simulink model "Sim_Multi"  (R2019b)
settings: Solver=VariableStepAuto  StartTime=0.0  StopTime=sim_time  FixedStep=t_sim  MaxStep=t_control  RelTol=1e-5  EnableMultiTasking=on
model workspace (MAT data in the model file):
  start_time = 1
values from neighbouring files (symbols this model uses):
  Att_init = [0;0;0] * d2r    [Init_Multi.m]
  Blade_flapping = 0    [Init_Multi.m]
  C_D = 0.40    (= 0.4)    [Init_Multi.m]
  CoG_nominal = [0;0;0.001]    [Init_Multi.m]
  CoG_real = [0;0;0.001]    [Init_Multi.m]
  Coriolis_correction = 0    [Init_Multi.m]
  d2r = pi/180    (= 0.0174532925199)    [Init_Multi.m]
  Dyn_thrust = 0    [Init_Multi.m]
  g = 9.80665    [Init_Multi.m]
  J_nominal = [Jxx Jxy Jxz;Jyx Jyy Jyz;Jzx Jzy Jzz]    [Init_Multi.m]
  J_real = [Jxx Jxy Jxz;Jyx Jyy Jyz;Jzx Jzy Jzz]    [Init_Multi.m]
  k1 = -1.125    [Init_Multi.m]
  k2 = -1.372    [Init_Multi.m]
  k3 = -1.718    [Init_Multi.m]
  k4 = -0.655    [Init_Multi.m]
  k_a1s = 1.5 / 4.0    (= 0.375)    [Init_Multi.m]
  k_beta = 0.23    [Init_Multi.m]
  kappa = 1.00    (= 1)    [Init_Multi.m]
  mass_nominal = 0.550    (= 0.55)    [Init_Multi.m]
  mass_real = 0.550    (= 0.55)    [Init_Multi.m]
  max_thrust = max_thrust + (MotorMatrix_nominal(i,7)*MotorMatrix_nominal(i,12)+MotorMatrix_nominal(i,8)*MotorMatrix_nominal(i,12)^2)    [Init_Multi.m]
  MaxRate_cmd = [360;360;120] * d2r    [Init_Multi.m]
  min_thrust = min_thrust + (MotorMatrix_nominal(i,7)*MotorMatrix_nominal(i,11)+MotorMatrix_nominal(i,8)*MotorMatrix_nominal(i,11)^2)    [Init_Multi.m]
  MotorMap = B' * inv(B * B')    [Init_Multi.m]
  MotorMatrix_nominal = [045 , 0.170 , -0.028 , -1 , 1.0 , 0.010 , [9.6820 , 0.010872]*1e-5 , [1.4504 , 0.0016312]*1e-6 , 0000 , 6000 , [0.0 , 0.0 , 0.0] , 8*2.54/100 , 11/1000;                         135 , 0.170 , -0.028 , +1 , 1.0 , 0.010 , [9.6820 , 0.010872]*1e-5 , [1.4504 , 0.0016312]*1e-6 , 0000 , 6000 , [0.0 , 0.0 , 0.0] , 8*2.54/100 , 11/1000;                         225 , 0.170 , -0.028 , -1 , 1.0 , 0.010 , [9. ...(+284 chars)    [Init_Multi.m]
  MotorMatrix_real = [045 , 0.170 , -0.028 , -1 , 1.0 , 0.010 , [9.6820 , 0.010872]*1e-5 , [1.4504 , 0.0016312]*1e-6 , 0000 , 6000 , [0.0 , 0.0 , 0.0] , 8*2.54/100 , 11/1000;                      135 , 0.170 , -0.028 , +1 , 1.0 , 0.010 , [9.6820 , 0.010872]*1e-5 , [1.4504 , 0.0016312]*1e-6 , 0000 , 6000 , [0.0 , 0.0 , 0.0] , 8*2.54/100 , 11/1000;                      225 , 0.170 , -0.028 , -1 , 1.0 , 0.010 , [9.6820 , ...(+275 chars)    [Init_Multi.m]
  Noise_flag = 1    [Init_Multi.m]
  omega_init = [0;0;0]    [Init_Multi.m]
  q_init = rpy2quat(Att_init)    [Init_Multi.m]
  r2d = 180/pi    (= 57.2957795131)    [Init_Multi.m]
  rho = 1.225    [Init_Multi.m]
  rpm2radpersec = 2*pi/60    (= 0.10471975512)    [Init_Multi.m]
  rpm_init = 3104.5025852    [Init_Multi.m]
  Surface_params = [a;b;c]    [Init_Multi.m]
  t_control = t_control_2*4    (= 0.02)    [Init_Multi.m]
  t_sim = 1/1000    (= 0.001)    [Init_Multi.m]
  thrust_reserve = 0.10    (= 0.1)    [Init_Multi.m]
  v_h = 4.0    (= 4)    [Init_Multi.m]
  Vb_init = [0;0;0]    [Init_Multi.m]
  Vi_init = R_IB_init' * Vb_init    [Init_Multi.m]
  Xi_init = [0;0;-1]    [Init_Multi.m]
undefined symbols (not defined in the file or in its folder): anti_windup_1, anti_windup_2, DiscIntNeverNeededParam, Kd_1, Kd_2, Kff_1, Kff_2, Ki_1, Ki_2, Kp_1, Kp_2, Kpass_1, magnitude, rpy2quat, thrust2rpm
libraries: simulink x35, dspsigops x3, sharedtransform x2, dspmtrx3 x1, robotuavlib x1, vrlib x1
(part 3 of 4)

== system Sim_Multi/Controller/Controller Structure/Pos//Vel Control/PI Rate controller1/Gain Kff ==
  Rate_cmd : Inport
  Constant1 : Constant  Value=Kff_1
  Create diagonal 3x3 matrix : Subsystem
  Product : Product  Multiplication=Matrix(*)  SampleTime=t_control  RndMeth=Zero
  Product1 : Product  Multiplication=Matrix(*)  RndMeth=Zero
  Out1 : Outport
  wires:
  [J_control] -> Product1/1
  Product1/1 -> Product/1
  Rate_cmd/1 -> Product/2
  Constant1/1 -> Create diagonal 3x3 matrix/1(Vector)
  Create diagonal 3x3 matrix/1(Matrix) -> Product1/2
  Product/1 -> Out1/1

== system Sim_Multi/Controller/Controller Structure/Pos//Vel Control/PI Rate controller1/Gain Ki ==
  Rate_error : Inport
  Constant1 : Constant  Value=Ki_1
  Create diagonal 3x3 matrix : Subsystem
  Product : Product  Multiplication=Matrix(*)  SampleTime=t_control  RndMeth=Zero
  Product1 : Product  Multiplication=Matrix(*)  RndMeth=Zero
  Out1 : Outport
  wires:
  [J_control] -> Product1/1
  Product1/1 -> Product/1
  Rate_error/1 -> Product/2
  Constant1/1 -> Create diagonal 3x3 matrix/1(Vector)
  Create diagonal 3x3 matrix/1(Matrix) -> Product1/2
  Product/1 -> Out1/1

== system Sim_Multi/Controller/Controller Structure/Pos//Vel Control/PI Rate controller1/Gain Kp ==
  Rate_error : Inport
  Constant1 : Constant  Value=Kp_1
  Create diagonal 3x3 matrix : Subsystem
  Product : Product  Multiplication=Matrix(*)  SampleTime=t_control  RndMeth=Zero
  Product1 : Product  Multiplication=Matrix(*)  RndMeth=Zero
  Out1 : Outport
  wires:
  [J_control] -> Product1/1
  Product1/1 -> Product/1
  Rate_error/1 -> Product/2
  Constant1/1 -> Create diagonal 3x3 matrix/1(Vector)
  Create diagonal 3x3 matrix/1(Matrix) -> Product1/2
  Product/1 -> Out1/1

== system Sim_Multi/Controller/Controller Structure/Pos//Vel Control/PID Attitude Controller (additionally controls altitude and yaw to take advantage of faster sampling rate)1/Gain Kd ==
  Rate_error : Inport
  Constant1 : Constant  Value=Kd_2
  Product : Product  RndMeth=Zero
  Out1 : Outport
  wires:
  Rate_error/1 -> Product/2
  Product/1 -> Out1/1
  Constant1/1 -> Product/1

== system Sim_Multi/Controller/Controller Structure/Pos//Vel Control/PID Attitude Controller (additionally controls altitude and yaw to take advantage of faster sampling rate)1/Gain Ki ==
  Rate_error : Inport
  Constant1 : Constant  Value=Ki_2
  Product : Product  RndMeth=Zero
  Out1 : Outport
  wires:
  Rate_error/1 -> Product/2
  Product/1 -> Out1/1
  Constant1/1 -> Product/1

== system Sim_Multi/Controller/Controller Structure/Pos//Vel Control/PID Attitude Controller (additionally controls altitude and yaw to take advantage of faster sampling rate)1/Gain Kp ==
  Rate_error : Inport
  Constant1 : Constant  Value=Kp_2
  Product : Product  RndMeth=Zero
  Out1 : Outport
  wires:
  Rate_error/1 -> Product/2
  Product/1 -> Out1/1
  Constant1/1 -> Product/1

== system Sim_Multi/Controller/Controller Structure/Pos//Vel Control/PID Position Controller (yaw and Z are passed though)1/Gain Kd ==
  Rate_error : Inport
  Constant1 : Constant  Value=Kd_1
  Product : Product  SampleTime=t_control  RndMeth=Zero
  Out1 : Outport
  wires:
  Rate_error/1 -> Product/2
  Product/1 -> Out1/1
  Constant1/1 -> Product/1

== system Sim_Multi/Controller/Controller Structure/Pos//Vel Control/PID Position Controller (yaw and Z are passed though)1/Gain Ki ==
  Rate_error : Inport
  Constant1 : Constant  Value=Ki_1
  Product : Product  SampleTime=t_control  RndMeth=Zero
  Out1 : Outport
  wires:
  Rate_error/1 -> Product/2
  Product/1 -> Out1/1
  Constant1/1 -> Product/1

== system Sim_Multi/Controller/Controller Structure/Pos//Vel Control/PID Position Controller (yaw and Z are passed though)1/Gain Kp ==
  Rate_error : Inport
  Constant1 : Constant  Value=Kp_1
  Product : Product  SampleTime=t_control  RndMeth=Zero
  Out1 : Outport
  wires:
  Rate_error/1 -> Product/2
  Product/1 -> Out1/1
  Constant1/1 -> Product/1

== system Sim_Multi/Plant/6DOF model/Calculate omega_dot/Cross Product omega x (J * omega)/Subsystem ==
  u : Inport
  v : Inport  Port=2
  Demux : Demux  Outputs=3
  Demux1 : Demux  Outputs=3
  Mux : Mux  Inputs=3
  Product : Product
  Product1 : Product
  Product2 : Product
  Positive elements : Outport
  wires:
  Mux/1 -> Positive elements/1
  v/1 -> Demux1/1
  u/1 -> Demux/1
  Demux/2 -> Product/1
  Demux1/3 -> Product/2
  Demux/3 -> Product1/1
  Demux1/1 -> Product1/2
  Demux/1 -> Product2/1
  Demux1/2 -> Product2/2
  Product/1 -> Mux/1  "u2*v3"
  Product1/1 -> Mux/2  "u3*v1"
  Product2/1 -> Mux/3  "u1*v2"

== system Sim_Multi/Plant/6DOF model/Calculate omega_dot/Cross Product omega x (J * omega)/Subsystem1 ==
  u : Inport
  v : Inport  Port=2
  Demux : Demux  Outputs=3
  Demux1 : Demux  Outputs=3
  Mux : Mux  Inputs=3
  Product : Product
  Product1 : Product
  Product2 : Product
  Negative elements : Outport
  wires:
  Mux/1 -> Negative elements/1
  v/1 -> Demux1/1
  u/1 -> Demux/1
  Product/1 -> Mux/1  "u3*v2"
  Product1/1 -> Mux/2  "u1*v3"
  Product2/1 -> Mux/3  "u2*v1"
  Demux/3 -> Product/1
  Demux1/2 -> Product/2
  Demux/1 -> Product1/1
  Demux1/3 -> Product1/2
  Demux/2 -> Product2/1
  Demux1/1 -> Product2/2

== system Sim_Multi/Plant/6DOF model/Quat Strapdown Eq./Cross Product/Subsystem ==
  u : Inport
  v : Inport  Port=2
  Demux : Demux  Outputs=3
  Demux1 : Demux  Outputs=3
  Mux : Mux  Inputs=3
  Product : Product
  Product1 : Product
  Product2 : Product
  Positive elements : Outport
  wires:
  Mux/1 -> Positive elements/1
  v/1 -> Demux1/1
  u/1 -> Demux/1
  Demux/2 -> Product/1
  Demux1/3 -> Product/2
  Demux/3 -> Product1/1
  Demux1/1 -> Product1/2
  Demux/1 -> Product2/1
  Demux1/2 -> Product2/2
  Product/1 -> Mux/1  "u2*v3"
  Product1/1 -> Mux/2  "u3*v1"
  Product2/1 -> Mux/3  "u1*v2"

== system Sim_Multi/Plant/6DOF model/Quat Strapdown Eq./Cross Product/Subsystem1 ==
  u : Inport
  v : Inport  Port=2
  Demux : Demux  Outputs=3
  Demux1 : Demux  Outputs=3
  Mux : Mux  Inputs=3
  Product : Product
  Product1 : Product
  Product2 : Product
  Negative elements : Outport
  wires:
  Mux/1 -> Negative elements/1
  v/1 -> Demux1/1
  u/1 -> Demux/1
  Product/1 -> Mux/1  "u3*v2"
  Product1/1 -> Mux/2  "u1*v3"
  Product2/1 -> Mux/3  "u2*v1"
  Demux/3 -> Product/1
  Demux1/2 -> Product/2
  Demux/1 -> Product1/1
  Demux1/3 -> Product1/2
  Demux/2 -> Product2/1
  Demux1/1 -> Product2/2

== system Sim_Multi/Plant/6DOF model/Quat Strapdown Eq./Normalize/norm ==
  u : Inport
  Complex to Real-Imag : ComplexToRealImag  Output=Real
  Sqrt : Sqrt  SaturateOnIntegerOverflow=on
  dot_product : Subsystem
  ||u|| : Outport
  wires:
  u/1 -> dot_product/1(u), dot_product/2(v)
  dot_product/1(u.v) -> Sqrt/1
  Sqrt/1 -> Complex to Real-Imag/1
  Complex to Real-Imag/1 -> ||u||/1

== system Sim_Multi/Plant/Force//Moment computation/Compute aerodynamic drag of the airframe in Body axes/Aerodynamic drag force/Nonzero airspeed ==
  Airspeed (Body) : Inport
  Surface_params : Inport  Port=2
  Action Port : ActionPort  ActionPortLabel=else
  Abs : Abs
  Constant : Constant  Value=1/2
  Constant1 : Constant  Value=rho
  Constant2 : Constant  Value=C_D
  Drag force opposes direction of airspeed : Gain  Gain=-1
  Normalize : Subsystem
  Product : Product  Inputs=5
  Product1 : Product
  Surface area computation : Subsystem
  u^2 : Subsystem
  Drag force : Outport
  wires:
  Airspeed (Body)/1 -> Surface area computation/1(Airspeed (Body)), Normalize/1(Input), u^2/1(u)
  Surface_params/1 -> Surface area computation/2(Surface_params)
  Constant/1 -> Product/1
  Constant1/1 -> Product/2
  u^2/1(u^2) -> Product/3
  Constant2/1 -> Product/4
  Surface area computation/1(Area) -> Product/5
  Normalize/1(Output) -> Product1/1  "Normalized airspeed vector (Body axes)"
  Product1/1 -> Drag force opposes direction of airspeed/1
  Drag force opposes direction of airspeed/1 -> Drag force/1
  Product/1 -> Abs/1
  Abs/1 -> Product1/2  "Magnitude of drag force"

== system Sim_Multi/Plant/Force//Moment computation/Compute aerodynamic drag of the airframe in Body axes/Aerodynamic drag force/Zero airspeed ==
  Airspeed : Inport
  Surface_params : Inport  Port=2
  Action Port : ActionPort  ActionPortLabel=if(u1 == 0)
  Constant : Constant  Value=[0;0;0]
  Terminator : Terminator
  Terminator1 : Terminator
  Drag force : Outport  InitialOutput=[0;0;-1]
  wires:
  Airspeed/1 -> Terminator/1  "Airspeed components in (unbent) rotor plane"
  Constant/1 -> Drag force/1
  Surface_params/1 -> Terminator1/1

== system Sim_Multi/Plant/Force//Moment computation/Compute aerodynamic drag of the airframe in Body axes/Aerodynamic drag force/norm ==
  u : Inport
  Complex to Real-Imag : ComplexToRealImag  Output=Real
  Sqrt : Sqrt  SaturateOnIntegerOverflow=on
  dot_product : Subsystem
  ||u|| : Outport
  wires:
  u/1 -> dot_product/1(u), dot_product/2(v)
  dot_product/1(u.v) -> Sqrt/1
  Sqrt/1 -> Complex to Real-Imag/1
  Complex to Real-Imag/1 -> ||u||/1

== system Sim_Multi/Plant/Force//Moment computation/Compute aerodynamic drag of the airframe in Body axes/Total airspeed (Body axes)/Inertial to Body ==
  DCM_ib : Inport
  Wind_i : Inport  Port=2
  Product : Product  Multiplication=Matrix(*)
  Reshape : Reshape  OutputDimensionality=Column vector (2-D)
  Reshape1 : Reshape  OutputDimensionality=Column vector (2-D)
  Wind_b : Outport
  wires:
  Reshape/1 -> Product/2
  Product/1 -> Reshape1/1
  Reshape1/1 -> Wind_b/1
  Wind_i/1 -> Reshape/1
  DCM_ib/1 -> Product/1  "DCM_ib"

== system Sim_Multi/Plant/Force//Moment computation/Forces and moments generated by spinning propellers/For Each Subsystem/Actuator dynamics ==
  note: This block diagram expresses the actuator dynamics of a specific motor/propeller combination
      | as a first order transfer function. The time constant and gain of this first order transfer function
      | for each motor is listed in the motor matrix.
      | In addition, upper and lower limits of the motor RPM can be set so that the motor output
      | never exceeds those values.
  MotorMatrix_real : Inport
  RPM_command : Inport  Port=2
  Continuous Integrator with dynamic upper/lower limits : Subsystem
  Divide : Product  Inputs=*/
  Product : Product  SampleTime=t_sim  RndMeth=Zero
  Rate Transition : RateTransition  OutPortSampleTime=t_sim
  Selector : Selector  InputPortWidth=17  IndexOptions=Index vector (dialog)  Indices=[5]  OutputSizes=1
  Selector1 : Selector  InputPortWidth=17  IndexOptions=Index vector (dialog)  Indices=[6]  OutputSizes=1
  Selector2 : Selector  InputPortWidth=17  IndexOptions=Index vector (dialog)  Indices=[11]  OutputSizes=1
  Selector3 : Selector  InputPortWidth=17  IndexOptions=Index vector (dialog)  Indices=[12]  OutputSizes=1
  Sum1 : Sum  Inputs=-+|
  RPM_motor : Outport
  wires:
  Sum1/1 -> Divide/1
  Selector1/1 -> Divide/2  "TF time constant"
  Product/1 -> Sum1/2
  Selector/1 -> Product/2  "TF gain"
  RPM_command/1 -> Product/1
  MotorMatrix_real/1 -> Selector3/1, Selector2/1, Selector1/1, Selector/1
  Divide/1 -> Continuous Integrator with dynamic upper/lower limits/1(Integrator input)
  Continuous Integrator with dynamic upper/lower limits/1(Output) -> Rate Transition/1, Sum1/1
  Selector2/1 -> Continuous Integrator with dynamic upper/lower limits/2(Lower limit)  "RPM min value"
  Selector3/1 -> Continuous Integrator with dynamic upper/lower limits/3(Upper limit)  "RPM max value"
  Rate Transition/1 -> RPM_motor/1

== system Sim_Multi/Plant/Force//Moment computation/Forces and moments generated by spinning propellers/For Each Subsystem/Cross Product ==
  r : Inport
  omega : Inport  Port=2
  Reshape : Reshape  OutputDimensionality=Column vector (2-D)
  Subsystem : Subsystem
  Subsystem1 : Subsystem
  Sum : Sum  Inputs=+|-
  omega x r : Outport
  wires:
  Sum/1 -> Reshape/1
  omega/1 -> Subsystem1/1(omega), Subsystem/1(omega)
  r/1 -> Subsystem1/2(r), Subsystem/2(r)
  Subsystem/1(Positive elements) -> Sum/1
  Subsystem1/1(Negative elements) -> Sum/2
  Reshape/1 -> omega x r/1

== system Sim_Multi/Plant/Force//Moment computation/Forces and moments generated by spinning propellers/For Each Subsystem/Leverarm vector from real CoG to each propeller (Body axes) ==
  note: This subsystem computes the leverarm vector from the real center of gravity
      | of the airframe to each propeller.
      | This vector is necessary to compute the moment contributions of each propeller.
  MotorMatrix_real : Inport
  CoG_real : Inport  Port=2
  Abs : Abs
  Conversion deg to rad : Gain  Gain=d2r
  Mux : Mux  Inputs=2
  Mux2 : Mux  Inputs=2
  Product4 : Product
  Reshape : Reshape  OutputDimensionality=Column vector (2-D)
  Reshape1 : Reshape  OutputDimensionality=Column vector (2-D)
  Selector3 : Selector  InputPortWidth=17  IndexOptions=Index vector (dialog)  Indices=[1]  OutputSizes=1
  Selector4 : Selector  InputPortWidth=17  IndexOptions=Index vector (dialog)  Indices=[2]  OutputSizes=1
  Selector5 : Selector  InputPortWidth=17  IndexOptions=Index vector (dialog)  Indices=[3]  OutputSizes=1
  Subtract : Sum  Inputs=+-
  Trigonometric Function : Trigonometry
  Trigonometric Function1 : Trigonometry  Operator=cos
  Prop_vector : Outport
  wires:
  Selector3/1 -> Conversion deg to rad/1  "Motor arm angle"
  Selector4/1 -> Abs/1  "Motor arm length"
  Selector5/1 -> Mux2/2  "Propeller Z offset"
  Conversion deg to rad/1 -> Trigonometric Function/1, Trigonometric Function1/1
  Trigonometric Function1/1 -> Mux/1  "Motor arm x component"
  Trigonometric Function/1 -> Mux/2  "Motor arm y component"
  Mux/1 -> Product4/1
  Abs/1 -> Product4/2
  Product4/1 -> Mux2/1  "Motor location x/y vector"
  Mux2/1 -> Reshape/1
  CoG_real/1 -> Reshape1/1  "Location of real CoG w.r.t. geometric center (Body axes)"
  Reshape/1 -> Subtract/1  "Vector from geometric center to propeller (Body axes)"
  Reshape1/1 -> Subtract/2
  Subtract/1 -> Prop_vector/1  "Vector from real CoG to propeller (Body axes)"
  MotorMatrix_real/1 -> Selector5/1, Selector4/1, Selector3/1

== system Sim_Multi/Plant/Force//Moment computation/Forces and moments generated by spinning propellers/For Each Subsystem/Thrust//moment vector for each propeller (Body axes) ==
  Prop_vector : Inport
  True airspeed : Inport  Port=2
  Body_rates : Inport  Port=3
  MotorMatrix_real : Inport  Port=4
  RPM_motor : Inport  Port=5
  6 DOF : Inport  Port=6
  Add : Sum  Inputs=++++
  Compute dynamic motor thrust and moments : Subsystem
  Coordinate transformation Body to Motor axes : Subsystem
  Cross Product : Subsystem
  Reshape : Reshape  OutputDimensionality=Column vector (2-D)
  Thrust_vector (Body axes) : Outport
  Motor_moments (Body axes) : Outport  Port=2
  wires:
  MotorMatrix_real/1 -> Coordinate transformation Body to Motor axes/1(MotorMatrix_real), Compute dynamic motor thrust and moments/2(MotorMatrix_real)
  True airspeed/1 -> Coordinate transformation Body to Motor axes/2(Airspeed (Body axes))
  Coordinate transformation Body to Motor axes/2(Airspeed (Motor axes)) -> Compute dynamic motor thrust and moments/4(Airspeed (Motor axes))
  RPM_motor/1 -> Compute dynamic motor thrust and moments/1(RPM_motor)
  Body_rates/1 -> Compute dynamic motor thrust and moments/5(Body_rates)
  Compute dynamic motor thrust and moments/3(Gyro moment (Body axes)) -> Add/3  "Gyroscopic moments per motor (Body axes)"
  Compute dynamic motor thrust and moments/1(Induced motor moment (Body axes)) -> Add/1  "Induced motor moment at dynamic conditions (Body axes)"
  Add/1 -> Motor_moments (Body axes)/1
  Coordinate transformation Body to Motor axes/1(R_mb) -> Compute dynamic motor thrust and moments/3(R_mb)
  Compute dynamic motor thrust and moments/4(Thrust_vector (Body axes)) -> Thrust_vector (Body axes)/1, Cross Product/2(v)
  Compute dynamic motor thrust and moments/2(Motor hub moment (Body axes)) -> Add/2  "Moment induced in motor hub due to blade flapping (Body axes)"
  Cross Product/1(u x v) -> Reshape/1
  Prop_vector/1 -> Cross Product/1(u)
  Reshape/1 -> Add/4
  6 DOF/1 -> Compute dynamic motor thrust and moments/6(6 DOF)

== system Sim_Multi/Plant/Force//Moment computation/Forces and moments generated by spinning propellers/Total airspeed (Body axes)/Inertial to Body ==
  DCM_ib : Inport
  Wind_i : Inport  Port=2
  Product : Product  Multiplication=Matrix(*)
  Reshape : Reshape  OutputDimensionality=Column vector (2-D)
  Reshape1 : Reshape  OutputDimensionality=Column vector (2-D)
  Wind_b : Outport
  wires:
  Reshape/1 -> Product/2
  Product/1 -> Reshape1/1
  Reshape1/1 -> Wind_b/1
  Wind_i/1 -> Reshape/1
  DCM_ib/1 -> Product/1  "DCM_ib"

== system Sim_Multi/State Estimation, Sensors, Noise/State estimation/Normalize/norm/dot_product ==
  u : Inport
  v : Inport  Port=2
  Product : Product  Multiplication=Matrix(*)  RndMeth=Zero
  Reshape : Reshape  OutputDimensionality=Column vector (2-D)
  Reshape1 : Reshape  OutputDimensionality=Column vector (2-D)
  transpose : Math  Operator=transpose  SaturateOnIntegerOverflow=on
  u.v : Outport
  wires:
  v/1 -> Reshape1/1
  u/1 -> Reshape/1
  Reshape/1 -> transpose/1
  transpose/1 -> Product/1
  Reshape1/1 -> Product/2
  Product/1 -> u.v/1

== system Sim_Multi/State Estimation, Sensors, Noise/State estimation/Normalize1/norm/dot_product ==
  u : Inport
  v : Inport  Port=2
  Product : Product  Multiplication=Matrix(*)  RndMeth=Zero
  Reshape : Reshape  OutputDimensionality=Column vector (2-D)
  Reshape1 : Reshape  OutputDimensionality=Column vector (2-D)
  transpose : Math  Operator=transpose  SaturateOnIntegerOverflow=on
  u.v : Outport
  wires:
  v/1 -> Reshape1/1
  u/1 -> Reshape/1
  Reshape/1 -> transpose/1
  transpose/1 -> Product/1
  Reshape1/1 -> Product/2
  Product/1 -> u.v/1

== system Sim_Multi/Controller/Controller Structure/Pos//Vel Control/PI Rate controller1/Cross Product/Subsystem ==
  u : Inport
  v : Inport  Port=2
  Demux : Demux  Outputs=3
  Demux1 : Demux  Outputs=3
  Mux : Mux  Inputs=3
  Product : Product
  Product1 : Product
  Product2 : Product
  Positive elements : Outport
  wires:
  Mux/1 -> Positive elements/1
  v/1 -> Demux1/1
  u/1 -> Demux/1
  Demux/2 -> Product/1
  Demux1/3 -> Product/2
  Demux/3 -> Product1/1
  Demux1/1 -> Product1/2
  Demux/1 -> Product2/1
  Demux1/2 -> Product2/2
  Product/1 -> Mux/1
  Product1/1 -> Mux/2
  Product2/1 -> Mux/3

== system Sim_Multi/Controller/Controller Structure/Pos//Vel Control/PI Rate controller1/Cross Product/Subsystem1 ==
  u : Inport
  v : Inport  Port=2
  Demux : Demux  Outputs=3
  Demux1 : Demux  Outputs=3
  Mux : Mux  Inputs=3
  Product : Product
  Product1 : Product
  Product2 : Product
  Negative elements : Outport
  wires:
  Mux/1 -> Negative elements/1
  v/1 -> Demux1/1
  u/1 -> Demux/1
  Product/1 -> Mux/1
  Product1/1 -> Mux/2
  Product2/1 -> Mux/3
  Demux/3 -> Product/1
  Demux1/2 -> Product/2
  Demux/1 -> Product1/1
  Demux1/3 -> Product1/2
  Demux/2 -> Product2/1
  Demux1/1 -> Product2/2

== system Sim_Multi/Controller/Controller Structure/Pos//Vel Control/PI Rate controller1/Gain Kff/Create diagonal 3x3 matrix ==
  Vector : Inport
  Constant2 : Constant  Value=0
  Demux : Demux  Outputs=3
  Subsystem9 : Subsystem
  Matrix : Outport
  wires:
  Demux/1 -> Subsystem9/1(C_11)
  Demux/2 -> Subsystem9/5(C_22)
  Vector/1 -> Demux/1
  Constant2/1 -> Subsystem9/8(C_32), Subsystem9/7(C_31), Subsystem9/6(C_23), Subsystem9/4(C_21), Subsystem9/3(C_13), Subsystem9/2(C_12)
  Subsystem9/1(Diag) -> Matrix/1
  Demux/3 -> Subsystem9/9(C_33)

== system Sim_Multi/Controller/Controller Structure/Pos//Vel Control/PI Rate controller1/Gain Ki/Create diagonal 3x3 matrix ==
  Vector : Inport
  Constant2 : Constant  Value=0
  Demux : Demux  Outputs=3
  Subsystem9 : Subsystem
  Matrix : Outport
  wires:
  Demux/1 -> Subsystem9/1(C_11)
  Demux/2 -> Subsystem9/5(C_22)
  Vector/1 -> Demux/1
  Constant2/1 -> Subsystem9/8(C_32), Subsystem9/7(C_31), Subsystem9/6(C_23), Subsystem9/4(C_21), Subsystem9/3(C_13), Subsystem9/2(C_12)
  Subsystem9/1(Diag) -> Matrix/1
  Demux/3 -> Subsystem9/9(C_33)

== system Sim_Multi/Controller/Controller Structure/Pos//Vel Control/PI Rate controller1/Gain Kp/Create diagonal 3x3 matrix ==
  Vector : Inport
  Constant2 : Constant  Value=0
  Demux : Demux  Outputs=3
  Subsystem9 : Subsystem
  Matrix : Outport
  wires:
  Demux/1 -> Subsystem9/1(C_11)
  Demux/2 -> Subsystem9/5(C_22)
  Vector/1 -> Demux/1
  Constant2/1 -> Subsystem9/8(C_32), Subsystem9/7(C_31), Subsystem9/6(C_23), Subsystem9/4(C_21), Subsystem9/3(C_13), Subsystem9/2(C_12)
  Subsystem9/1(Diag) -> Matrix/1
  Demux/3 -> Subsystem9/9(C_33)

== system Sim_Multi/Plant/6DOF model/Quat Strapdown Eq./Normalize/norm/dot_product ==
  u : Inport
  v : Inport  Port=2
  Product : Product  Multiplication=Matrix(*)  RndMeth=Zero
  Reshape : Reshape  OutputDimensionality=Column vector (2-D)
  Reshape1 : Reshape  OutputDimensionality=Column vector (2-D)
  transpose : Math  Operator=transpose  SaturateOnIntegerOverflow=on
  u.v : Outport
  wires:
  v/1 -> Reshape1/1
  u/1 -> Reshape/1
  Reshape/1 -> transpose/1
  transpose/1 -> Product/1
  Reshape1/1 -> Product/2
  Product/1 -> u.v/1

== system Sim_Multi/Plant/Force//Moment computation/Compute aerodynamic drag of the airframe in Body axes/Aerodynamic drag force/Nonzero airspeed/Normalize ==
  Input : Inport
  Divide : Product  Inputs=*/
  norm : Subsystem
  Output : Outport
  wires:
  Input/1 -> Divide/1, norm/1(u)
  norm/1(||u||) -> Divide/2
  Divide/1 -> Output/1

== system Sim_Multi/Plant/Force//Moment computation/Compute aerodynamic drag of the airframe in Body axes/Aerodynamic drag force/Nonzero airspeed/Surface area computation ==
  Airspeed (Body) : Inport
  Surface_params : Inport  Port=2
  Scaling factor computation : Subsystem
  Surface area computation : Subsystem
  Area : Outport
  wires:
  Surface_params/1 -> Scaling factor computation/2(Surface_params)
  Airspeed (Body)/1 -> Surface area computation/1(Airspeed (Body)), Scaling factor computation/1(Airspeed (Body))
  Scaling factor computation/1(Scaling factor) -> Surface area computation/2(Scaling factor)
  Surface area computation/1(Surface area) -> Area/1

== system Sim_Multi/Plant/Force//Moment computation/Compute aerodynamic drag of the airframe in Body axes/Aerodynamic drag force/Nonzero airspeed/u^2 ==
  u : Inport
  dot_product : Subsystem
  u^2 : Outport
  wires:
  u/1 -> dot_product/1(u), dot_product/2(v)
  dot_product/1(u.v) -> u^2/1

== system Sim_Multi/Plant/Force//Moment computation/Compute aerodynamic drag of the airframe in Body axes/Aerodynamic drag force/norm/dot_product ==
  u : Inport
  v : Inport  Port=2
  Product : Product  Multiplication=Matrix(*)  RndMeth=Zero
  Reshape : Reshape  OutputDimensionality=Column vector (2-D)
  Reshape1 : Reshape  OutputDimensionality=Column vector (2-D)
  transpose : Math  Operator=transpose  SaturateOnIntegerOverflow=on
  u.v : Outport
  wires:
  v/1 -> Reshape1/1
  u/1 -> Reshape/1
  Reshape/1 -> transpose/1
  transpose/1 -> Product/1
  Reshape1/1 -> Product/2
  Product/1 -> u.v/1

== system Sim_Multi/Plant/Force//Moment computation/Forces and moments generated by spinning propellers/For Each Subsystem/Actuator dynamics/Continuous Integrator with dynamic upper//lower limits ==
  Integrator input : Inport
  Lower limit : Inport  Port=2
  Upper limit : Inport  Port=3
  Compare To Zero : simulink/Logic and Bit Operations/Compare To Zero  relop=<  OutDataTypeStr=uint8  ZeroCross=off
  Compare To Zero1 : simulink/Logic and Bit Operations/Compare To Zero  relop=>  OutDataTypeStr=uint8  ZeroCross=off
  Constant : Constant  Value=0
  Integrator : Integrator  InitialCondition=rpm_init
  Logical Operator : Logic  Operator=OR  AllPortsSameDT=off  OutDataTypeStr=boolean
  Logical Operator1 : Logic  Operator=OR  AllPortsSameDT=off  OutDataTypeStr=boolean
  Logical Operator2 : Logic  AllPortsSameDT=off  OutDataTypeStr=boolean
  Relational Operator : RelationalOperator  Operator=<=  OutDataTypeStr=boolean  RndMeth=Nearest
  Relational Operator1 : RelationalOperator  OutDataTypeStr=boolean  RndMeth=Nearest
  Saturation Dynamic : simulink/Discontinuities/Saturation Dynamic  OutMin=[]  OutMax=[]  OutDataTypeStr=Inherit: Same as second input  OutDataType=fixdt(1, 16)  OutScaling=2^-10  DoSatur=off
  Switch : Switch  Criteria=u2 > Threshold
  Output : Outport
  wires:
  Integrator input/1 -> Switch/1, Compare To Zero1/1, Compare To Zero/1
  Constant/1 -> Switch/3
  Switch/1 -> Integrator/1
  Relational Operator/1 -> Logical Operator/1
  Compare To Zero/1 -> Logical Operator/2
  Upper limit/1 -> Relational Operator/2, Saturation Dynamic/1
  Lower limit/1 -> Saturation Dynamic/3, Relational Operator1/2
  Compare To Zero1/1 -> Logical Operator1/1
  Relational Operator1/1 -> Logical Operator1/2
  Logical Operator1/1 -> Logical Operator2/2
  Logical Operator/1 -> Logical Operator2/1
  Logical Operator2/1 -> Switch/2
  Saturation Dynamic/1 -> Output/1
  Integrator/1 -> Relational Operator/1, Saturation Dynamic/2, Relational Operator1/1

== system Sim_Multi/Plant/Force//Moment computation/Forces and moments generated by spinning propellers/For Each Subsystem/Cross Product/Subsystem ==
  omega : Inport
  r : Inport  Port=2
  Demux : Demux  Outputs=3
  Demux1 : Demux  Outputs=3
  Mux : Mux  Inputs=3
  Product : Product
  Product1 : Product
  Product2 : Product
  Positive elements : Outport
  wires:
  Mux/1 -> Positive elements/1
  r/1 -> Demux1/1
  omega/1 -> Demux/1
  Demux/2 -> Product/1
  Demux1/3 -> Product/2
  Demux/3 -> Product1/1
  Demux1/1 -> Product1/2
  Demux/1 -> Product2/1
  Demux1/2 -> Product2/2
  Product/1 -> Mux/1  "u2*v3"
  Product1/1 -> Mux/2  "u3*v1"
  Product2/1 -> Mux/3  "u1*v2"

== system Sim_Multi/Plant/Force//Moment computation/Forces and moments generated by spinning propellers/For Each Subsystem/Cross Product/Subsystem1 ==
  omega : Inport
  r : Inport  Port=2
  Demux : Demux  Outputs=3
  Demux1 : Demux  Outputs=3
  Mux : Mux  Inputs=3
  Product : Product
  Product1 : Product
  Product2 : Product
  Negative elements : Outport
  wires:
  Mux/1 -> Negative elements/1
  r/1 -> Demux1/1
  omega/1 -> Demux/1
  Product/1 -> Mux/1  "u3*v2"
  Product1/1 -> Mux/2  "u1*v3"
  Product2/1 -> Mux/3  "u2*v1"
  Demux/3 -> Product/1
  Demux1/2 -> Product/2
  Demux/1 -> Product1/1
  Demux1/3 -> Product1/2
  Demux/2 -> Product2/1
  Demux1/1 -> Product2/2

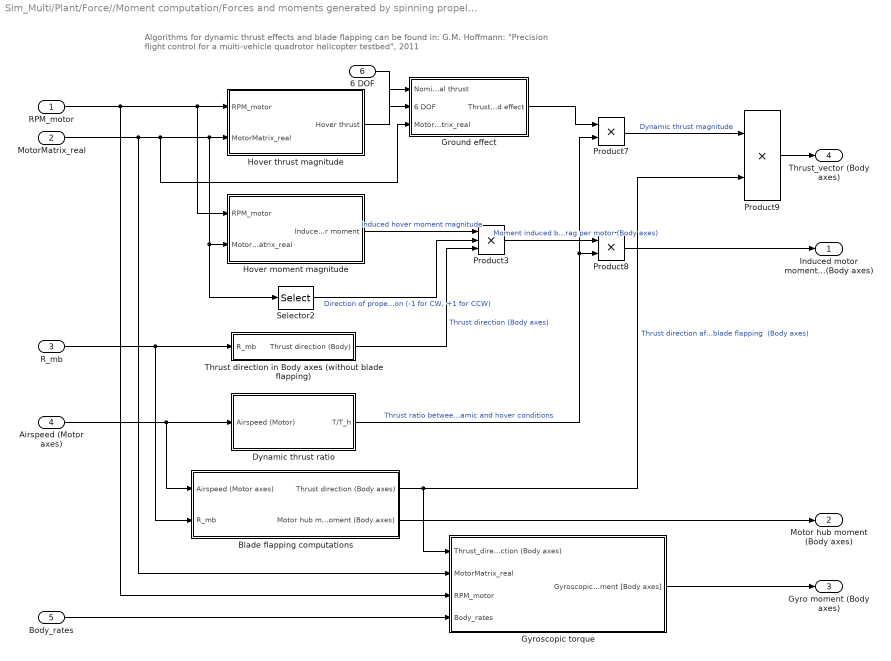
== system Sim_Multi/Plant/Force//Moment computation/Forces and moments generated by spinning propellers/For Each Subsystem/Thrust//moment vector for each propeller (Body axes)/Compute dynamic motor thrust and moments ==
  note: Algorithms for dynamic thrust effects and blade flapping can be found in:
      | G.M. Hoffmann: "Precision flight control for a multi-vehicle quadrotor helicopter testbed", 2011
  RPM_motor : Inport
  MotorMatrix_real : Inport  Port=2
  R_mb : Inport  Port=3
  Airspeed (Motor axes) : Inport  Port=4
  Body_rates : Inport  Port=5
  6 DOF : Inport  Port=6
  Blade flapping computations : Subsystem
  Dynamic thrust ratio : Subsystem
  Ground effect : Subsystem
  Gyroscopic torque : Subsystem
  Hover moment magnitude : Subsystem
  Hover thrust magnitude : Subsystem
  Product3 : Product  Inputs=3
  Product7 : Product
  Product8 : Product
  Product9 : Product
  Selector2 : Selector  InputPortWidth=17  IndexOptions=Index vector (dialog)  Indices=[4]  OutputSizes=1
  Thrust direction in Body axes (without blade flapping) : Subsystem
  Induced motor moment (Body axes) : Outport
  Motor hub moment (Body axes) : Outport  Port=2
  Gyro moment (Body axes) : Outport  Port=3
  Thrust_vector (Body axes) : Outport  Port=4
  wires:
  RPM_motor/1 -> Gyroscopic torque/3(RPM_motor), Hover moment magnitude/1(RPM_motor), Hover thrust magnitude/1(RPM_motor)
  MotorMatrix_real/1 -> Gyroscopic torque/2(MotorMatrix_real), Ground effect/3(MotorMatrix_real), Selector2/1, Hover moment magnitude/2(MotorMatrix_real), Hover thrust magnitude/2(MotorMatrix_real)
  Selector2/1 -> Product3/2  "Direction of propeller rotation (-1 for CW, +1 for CCW)"
  Thrust direction in Body axes (without blade flapping)/1(Thrust direction (Body)) -> Product3/3  "Thrust direction (Body axes)"
  R_mb/1 -> Blade flapping computations/2(R_mb), Thrust direction in Body axes (without blade flapping)/1(R_mb)
  Airspeed (Motor axes)/1 -> Blade flapping computations/1(Airspeed (Motor axes)), Dynamic thrust ratio/1(Airspeed (Motor))
  Product3/1 -> Product8/1  "Moment induced by aerodynamic drag per motor (Body axes)"
  Product8/1 -> Induced motor moment (Body axes)/1
  Product7/1 -> Product9/1  "Dynamic thrust magnitude"
  Product9/1 -> Thrust_vector (Body axes)/1
  Blade flapping computations/1(Thrust direction (Body axes)) -> Gyroscopic torque/1(Thrust_direction (Body axes)), Product9/2  "Thrust direction after blade flapping  (Body axes)"
  Blade flapping computations/2(Motor hub moment (Body axes)) -> Motor hub moment (Body axes)/1
  Body_rates/1 -> Gyroscopic torque/4(Body_rates)
  Gyroscopic torque/1(Gyroscopic moment [Body axes]) -> Gyro moment (Body axes)/1
  Hover thrust magnitude/1(Hover thrust) -> Ground effect/1(Nominal thrust)
  Hover moment magnitude/1(Induced hover moment) -> Product3/1  "Induced hover moment magnitude"
  Dynamic thrust ratio/1(T/T_h) -> Product7/2, Product8/2  "Thrust ratio between dynamic and hover conditions"
  Ground effect/1(Thrust with ground effect) -> Product7/1
  6 DOF/1 -> Ground effect/2(6 DOF)

== system Sim_Multi/Plant/Force//Moment computation/Forces and moments generated by spinning propellers/For Each Subsystem/Thrust//moment vector for each propeller (Body axes)/Coordinate transformation Body to Motor axes ==
  note: The true airspeed at prop computed here is the linear velocity (now in Motor axes)
      | with which this particular motor moves through the air.
      | So the point of view is: the surrounding air standing still and the airframe moving through it.
  MotorMatrix_real : Inport
  Airspeed (Body axes) : Inport  Port=2
  Conversion deg to rad : Gain  Gain=d2r
  Product : Product  Multiplication=Matrix(*)
  Rotation Matrix Body to Motor : Subsystem
  Selector : Selector  InputPortWidth=17  IndexOptions=Index vector (dialog)  Indices=[13 14 15]  OutputSizes=1
  R_mb : Outport
  Airspeed (Motor axes) : Outport  Port=2
  wires:
  Product/1 -> Airspeed (Motor axes)/1  "True airspeed at prop (Motor axes)"
  Rotation Matrix Body to Motor/1(R_mb) -> R_mb/1, Product/1  "Rotation matrix Body to Motor axes"
  MotorMatrix_real/1 -> Selector/1
  Selector/1 -> Conversion deg to rad/1
  Airspeed (Body axes)/1 -> Product/2  "True airspeed at prop (Body axes)"
  Conversion deg to rad/1 -> Rotation Matrix Body to Motor/1(Motor angles)

== system Sim_Multi/Plant/Force//Moment computation/Forces and moments generated by spinning propellers/For Each Subsystem/Thrust//moment vector for each propeller (Body axes)/Cross Product ==
  u : Inport
  v : Inport  Port=2
  Subsystem : Subsystem
  Subsystem1 : Subsystem
  Sum : Sum  Inputs=+|-
  u x v : Outport
  wires:
  Sum/1 -> u x v/1
  u/1 -> Subsystem1/1(u), Subsystem/1(u)
  v/1 -> Subsystem1/2(v), Subsystem/2(v)
  Subsystem/1(Positive elements) -> Sum/1
  Subsystem1/1(Negative elements) -> Sum/2

== system Sim_Multi/Controller/Controller Structure/Pos//Vel Control/PI Rate controller1/Gain Kff/Create diagonal 3x3 matrix/Subsystem9 ==
  C_11 : Inport  PortDimensions=1
  C_12 : Inport  Port=2  PortDimensions=1
  C_13 : Inport  Port=3  PortDimensions=1
  C_21 : Inport  Port=4  PortDimensions=1
  C_22 : Inport  Port=5  PortDimensions=1
  C_23 : Inport  Port=6  PortDimensions=1
  C_31 : Inport  Port=7  PortDimensions=1
  C_32 : Inport  Port=8  PortDimensions=1
  C_33 : Inport  Port=9  PortDimensions=1
  Reshape (9) to [3x3] column-major : Reshape  OutputDimensionality=Customize  OutputDimensions=[3,3]
  Vector Concatenate : Concatenate  NumInputs=9
  Diag : Outport
  wires:
  C_33/1 -> Vector Concatenate/9
  C_22/1 -> Vector Concatenate/5
  Reshape (9) to [3x3] column-major/1 -> Diag/1
  C_11/1 -> Vector Concatenate/1
  Vector Concatenate/1 -> Reshape (9) to [3x3] column-major/1
  C_32/1 -> Vector Concatenate/6
  C_31/1 -> Vector Concatenate/3
  C_21/1 -> Vector Concatenate/2
  C_13/1 -> Vector Concatenate/7
  C_12/1 -> Vector Concatenate/4
  C_23/1 -> Vector Concatenate/8

== system Sim_Multi/Controller/Controller Structure/Pos//Vel Control/PI Rate controller1/Gain Ki/Create diagonal 3x3 matrix/Subsystem9 ==
  C_11 : Inport  PortDimensions=1
  C_12 : Inport  Port=2  PortDimensions=1
  C_13 : Inport  Port=3  PortDimensions=1
  C_21 : Inport  Port=4  PortDimensions=1
  C_22 : Inport  Port=5  PortDimensions=1
  C_23 : Inport  Port=6  PortDimensions=1
  C_31 : Inport  Port=7  PortDimensions=1
  C_32 : Inport  Port=8  PortDimensions=1
  C_33 : Inport  Port=9  PortDimensions=1
  Reshape (9) to [3x3] column-major : Reshape  OutputDimensionality=Customize  OutputDimensions=[3,3]
  Vector Concatenate : Concatenate  NumInputs=9
  Diag : Outport
  wires:
  C_33/1 -> Vector Concatenate/9
  C_22/1 -> Vector Concatenate/5
  Reshape (9) to [3x3] column-major/1 -> Diag/1
  C_11/1 -> Vector Concatenate/1
  Vector Concatenate/1 -> Reshape (9) to [3x3] column-major/1
  C_32/1 -> Vector Concatenate/6
  C_31/1 -> Vector Concatenate/3
  C_21/1 -> Vector Concatenate/2
  C_13/1 -> Vector Concatenate/7
  C_12/1 -> Vector Concatenate/4
  C_23/1 -> Vector Concatenate/8

== system Sim_Multi/Controller/Controller Structure/Pos//Vel Control/PI Rate controller1/Gain Kp/Create diagonal 3x3 matrix/Subsystem9 ==
  C_11 : Inport  PortDimensions=1
  C_12 : Inport  Port=2  PortDimensions=1
  C_13 : Inport  Port=3  PortDimensions=1
  C_21 : Inport  Port=4  PortDimensions=1
  C_22 : Inport  Port=5  PortDimensions=1
  C_23 : Inport  Port=6  PortDimensions=1
  C_31 : Inport  Port=7  PortDimensions=1
  C_32 : Inport  Port=8  PortDimensions=1
  C_33 : Inport  Port=9  PortDimensions=1
  Reshape (9) to [3x3] column-major : Reshape  OutputDimensionality=Customize  OutputDimensions=[3,3]
  Vector Concatenate : Concatenate  NumInputs=9
  Diag : Outport
  wires:
  C_33/1 -> Vector Concatenate/9
  C_22/1 -> Vector Concatenate/5
  Reshape (9) to [3x3] column-major/1 -> Diag/1
  C_11/1 -> Vector Concatenate/1
  Vector Concatenate/1 -> Reshape (9) to [3x3] column-major/1
  C_32/1 -> Vector Concatenate/6
  C_31/1 -> Vector Concatenate/3
  C_21/1 -> Vector Concatenate/2
  C_13/1 -> Vector Concatenate/7
  C_12/1 -> Vector Concatenate/4
  C_23/1 -> Vector Concatenate/8

== system Sim_Multi/Plant/Force//Moment computation/Compute aerodynamic drag of the airframe in Body axes/Aerodynamic drag force/Nonzero airspeed/Normalize/norm ==
  u : Inport
  Complex to Real-Imag : ComplexToRealImag  Output=Real
  Sqrt : Sqrt  SaturateOnIntegerOverflow=on
  dot_product : Subsystem
  ||u|| : Outport
  wires:
  u/1 -> dot_product/1(u), dot_product/2(v)
  dot_product/1(u.v) -> Sqrt/1
  Sqrt/1 -> Complex to Real-Imag/1
  Complex to Real-Imag/1 -> ||u||/1

== system Sim_Multi/Plant/Force//Moment computation/Compute aerodynamic drag of the airframe in Body axes/Aerodynamic drag force/Nonzero airspeed/Surface area computation/Scaling factor computation ==
  Airspeed (Body) : Inport
  Surface_params : Inport  Port=2
  Add : Sum  Inputs=+++
  Demux : Demux  Outputs=3
  Demux1 : Demux  Outputs=3
  Divide : Product  Inputs=*/
  Divide1 : Product  Inputs=*/
  Divide2 : Product  Inputs=*/
  Product : Product
  Product1 : Product
  Product2 : Product
  Reciprocal Sqrt : Sqrt  Operator=rSqrt  SaturateOnIntegerOverflow=on
  Scaling factor : Outport
  wires:
  Divide2/1 -> Product2/2, Product2/1
  Reciprocal Sqrt/1 -> Scaling factor/1
  Demux1/3 -> Divide2/2  "c"
  Demux/3 -> Divide2/1  "z"
  Divide/1 -> Product/2, Product/1
  Airspeed (Body)/1 -> Demux/1
  Surface_params/1 -> Demux1/1
  Demux1/1 -> Divide/2  "a"
  Demux/1 -> Divide/1  "x"
  Product/1 -> Add/1
  Product2/1 -> Add/3
  Add/1 -> Reciprocal Sqrt/1
  Demux/2 -> Divide1/1  "y"
  Divide1/1 -> Product1/2, Product1/1
  Demux1/2 -> Divide1/2  "b"
  Product1/1 -> Add/2

== system Sim_Multi/Plant/Force//Moment computation/Compute aerodynamic drag of the airframe in Body axes/Aerodynamic drag force/Nonzero airspeed/Surface area computation/Surface area computation ==
  Airspeed (Body) : Inport
  Scaling factor : Inport  Port=2
  Product : Product
  norm : Subsystem
  Surface area : Outport
  wires:
  Scaling factor/1 -> Product/2
  Airspeed (Body)/1 -> Product/1
  Product/1 -> norm/1(u)
  norm/1(||u||) -> Surface area/1

== system Sim_Multi/Plant/Force//Moment computation/Compute aerodynamic drag of the airframe in Body axes/Aerodynamic drag force/Nonzero airspeed/u^2/dot_product ==
  u : Inport
  v : Inport  Port=2
  Product : Product  Multiplication=Matrix(*)  RndMeth=Zero
  Reshape : Reshape  OutputDimensionality=Column vector (2-D)
  Reshape1 : Reshape  OutputDimensionality=Column vector (2-D)
  transpose : Math  Operator=transpose  SaturateOnIntegerOverflow=on
  u.v : Outport
  wires:
  v/1 -> Reshape1/1
  u/1 -> Reshape/1
  Reshape/1 -> transpose/1
  transpose/1 -> Product/1
  Reshape1/1 -> Product/2
  Product/1 -> u.v/1

== system Sim_Multi/Plant/Force//Moment computation/Forces and moments generated by spinning propellers/For Each Subsystem/Thrust//moment vector for each propeller (Body axes)/Compute dynamic motor thrust and moments/Blade flapping computations ==
  note: Blade flapping computations are motivated by algorithms found in:
      | G.M. Hoffmann: "Precision flight control for a multi-vehicle quadrotor helicopter testbed", 2011
      | The idea is the following:
      | The thrust vector is tilted backwards from the direction of motion. The amount of tilt depends on the magnitude of the airspeed vector in the (untilted) propeller plane.
      | The tilt direction is in the plane defined by the airspeed xy vector and the (untilted) thrust vector in Motor axes.
      | The normal vector to this plane can be found by computing the cross product of untilted thrust vector and airspeed xy vector.
      | The new (tilted) thrust vector can then be found by applying the Rodrigues rotation formula, see Wikipedia
  Airspeed (Motor axes) : Inport
  R_mb : Inport  Port=2
  Demux4 : Demux  Outputs=[2,1]
  If : If  IfExpression=u1 == 0
  Merge : Merge
  Merge1 : Merge
  Nonzero airspeed in rotor plane : Subsystem  TreatAsAtomicUnit=on
  Terminator : Terminator
  Zero airspeed in rotor plane : Subsystem  TreatAsAtomicUnit=on
  norm : Subsystem
  Thrust direction (Body axes) : Outport
  Motor hub moment (Body axes) : Outport  Port=2
  wires:
  If/1 -> Zero airspeed in rotor plane/Action
  Zero airspeed in rotor plane/1(Thrust direction (Body)) -> Merge/1
  Nonzero airspeed in rotor plane/1(Thrust direction (Body)) -> Merge/2
  If/2 -> Nonzero airspeed in rotor plane/Action
  Airspeed (Motor axes)/1 -> Demux4/1
  Demux4/2 -> Terminator/1  "Airspeed component along motor shaft"
  Demux4/1 -> norm/1(u), Zero airspeed in rotor plane/1(Airspeed xy), Nonzero airspeed in rotor plane/1(Airspeed xy)  "Airspeed components in (unbent) rotor plane"
  norm/1(||u||) -> If/1  "Airspeed xy component  magnitude"
  Merge/1 -> Thrust direction (Body axes)/1  "New tilted thrust direction (Body axes) (This is a unit vector)"
  R_mb/1 -> Nonzero airspeed in rotor plane/2(R_mb), Zero airspeed in rotor plane/2(R_mb)
  Merge1/1 -> Motor hub moment (Body axes)/1  "Moment in the motor hub due to bending of the propeller (Body axes)"
  Zero airspeed in rotor plane/2(Hub moment (Body)) -> Merge1/1
  Nonzero airspeed in rotor plane/2(Hub moment (Body)) -> Merge1/2

== system Sim_Multi/Plant/Force//Moment computation/Forces and moments generated by spinning propellers/For Each Subsystem/Thrust//moment vector for each propeller (Body axes)/Compute dynamic motor thrust and moments/Dynamic thrust ratio ==
  Airspeed (Motor) : Inport
  Angle of attack and airspeed magnitude : Subsystem
  Compute the climb speed : Subsystem
  Constant : Constant
  Constant1 : Constant  Value=Dyn_thrust
  Divide : Product  Inputs=*/
  Flight modes of the propeller : Subsystem
  Induced velocity at hover : Constant  Value=v_h
  Product2 : Product
  Sum2 : Sum  Inputs=|+-
  Switch : Switch  Criteria=u2 > Threshold  Threshold=0.5
  Trigonometric Function : Trigonometry
  T/T_h : Outport
  wires:
  Airspeed (Motor)/1 -> Angle of attack and airspeed magnitude/1(Airspeed (Motor axes)), Compute the climb speed/1(Airspeed (Motor axes))
  Trigonometric Function/1 -> Product2/1
  Sum2/1 -> Divide/2
  Angle of attack and airspeed magnitude/2(Airspeed magnitude) -> Product2/2  "Airspeed magnitude v_inf"
  Angle of attack and airspeed magnitude/1(AoA (rad)) -> Trigonometric Function/1  "Angle of Attack"
  Compute the climb speed/1(v_c) -> Flight modes of the propeller/2(v_c)
  Flight modes of the propeller/1(v_i) -> Sum2/1
  Product2/1 -> Sum2/2
  Induced velocity at hover/1 -> Divide/1, Flight modes of the propeller/1(v_h)
  Switch/1 -> T/T_h/1  "Thrust ratio T/T_h"
  Divide/1 -> Switch/1
  Constant/1 -> Switch/3
  Constant1/1 -> Switch/2

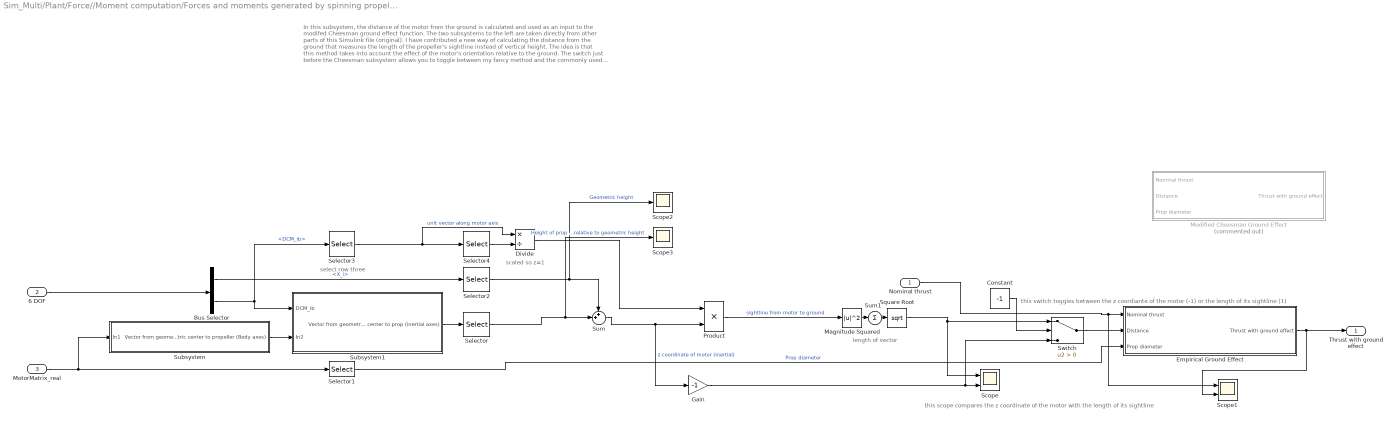
== system Sim_Multi/Plant/Force//Moment computation/Forces and moments generated by spinning propellers/For Each Subsystem/Thrust//moment vector for each propeller (Body axes)/Compute dynamic motor thrust and moments/Ground effect ==
  note: length of vector
  note: In this subsystem, the distance of the motor from the ground is calculated and used as an input to the modifed Cheesman ground effect function.
      |
      | The two subsystems to the left are taken directly from other parts of this Simulink file (original).
      |
      | I have contributed a new way of calculating the distance from the ground that measures the length of the propeller's sightline instead of vertical height.
      | The idea is that this method takes into account the effect of the motor's orientation relative to the ground.
      | The switch just before the Cheesman subsystem allows you to toggle between my fancy method and the commonly used height value.
  note: this switch toggles between the z coordiante of the motor (-1) or the length of its sightline (1)
  note: this scope compares the z coordinate of the motor with the length of its sightline
  note: scaled so z=1
  note: select row three
  Nominal thrust : Inport
  6 DOF : Inport  Port=2
  MotorMatrix_real : Inport  Port=3
  Bus Selector : BusSelector  OutputSignals=X_i,DCM_ib
  Constant : Constant  Value=-1
  Divide : Product  Inputs=*/
  Empirical Ground Effect : Subsystem
  Gain : Gain  Gain=-1
  Magnitude Squared : Math  Operator=magnitude^2  SignedPower=off  SaturateOnIntegerOverflow=on
  Modified Cheesman Ground Effect : Subsystem  Commented=on
  Product : Product
  Scope : Scope  NumInputPorts=2
  Scope1 : Scope  NumInputPorts=2
  Scope2 : Scope
  Scope3 : Scope
  Selector : Selector  InputPortWidth=3  IndexOptions=Index vector (dialog)  Indices=[3]  OutputSizes=1
  Selector1 : Selector  InputPortWidth=17  IndexOptions=Index vector (dialog)  Indices=[16]  OutputSizes=1
  Selector2 : Selector  InputPortWidth=3  IndexOptions=Index vector (dialog)  Indices=[3]  OutputSizes=1
  Selector3 : Selector  NumberOfDimensions=2  InputPortWidth=9  IndexOptions=Index vector (dialog),Select all  Indices=3,1  OutputSizes=1,1
  Selector4 : Selector  InputPortWidth=3  IndexOptions=Index vector (dialog)  Indices=[3]  OutputSizes=1
  Square Root : Sqrt  SaturateOnIntegerOverflow=on
  Subsystem : Subsystem
  Subsystem1 : Subsystem
  Sum : Sum  Inputs=++|
  Sum1 : Sum  Inputs=|+|
  Switch : Switch  Criteria=u2 > Threshold
  Thrust with ground effect : Outport
  wires:
  Selector4/1 -> Divide/2
  Nominal thrust/1 -> Scope1/1, Empirical Ground Effect/1(Nominal thrust)
  Divide/1 -> Product/1
  Selector2/1 -> Scope2/1, Sum/1  "Geometric height"
  MotorMatrix_real/1 -> Subsystem/1(In1), Selector1/1
  Bus Selector/1 -> Selector2/1  "<X_i>"
  Sum1/1 -> Square Root/1
  Magnitude Squared/1 -> Sum1/1
  Selector/1 -> Scope3/1, Sum/2  "Height of prop relative to geometric height"
  Subsystem1/1(Vector from geometric center to prop (inertial axes)) -> Selector/1
  6 DOF/1 -> Bus Selector/1
  Product/1 -> Magnitude Squared/1  "sightline from motor to ground"
  Empirical Ground Effect/1(Thrust with ground effect) -> Scope1/2, Thrust with ground effect/1
  Selector1/1 -> Empirical Ground Effect/3(Prop diameter)  "Prop diameter"
  Subsystem/1(Vector from geometric center to propeller (Body axes)) -> Subsystem1/2(In2)
  Selector3/1 -> Selector4/1, Divide/1  "unit vector along motor axis"
  Bus Selector/2 -> Selector3/1, Subsystem1/1(DCM_ib)  "<DCM_ib>"
  Sum/1 -> Gain/1, Product/2  "z coordinate of motor (inertial)"
  Switch/1 -> Empirical Ground Effect/2(Distance)
  Square Root/1 -> Scope/1, Switch/1
  Constant/1 -> Switch/2
  Gain/1 -> Switch/3, Scope/2

== system Sim_Multi/Plant/Force//Moment computation/Forces and moments generated by spinning propellers/For Each Subsystem/Thrust//moment vector for each propeller (Body axes)/Compute dynamic motor thrust and moments/Gyroscopic torque ==
  note: The thrust direction chosen here is the one after the effects of blade flapping.
      | The reasoning being that the propeller is bent in that direction and therefore
      | a majority of its moment of inertia effects will act in that direction as well (even
      | though the motor is not affected by blade flapping).
  Thrust_direction (Body axes) : Inport
  MotorMatrix_real : Inport  Port=2
  RPM_motor : Inport  Port=3
  Body_rates : Inport  Port=4
  Conversion rpm to rad/s : Gain  Gain=rpm2radpersec
  Cross Product : Subsystem
  Product5 : Product  Inputs=4
  Propeller moment of inertia : Subsystem
  Reshape1 : Reshape  OutputDimensionality=Column vector (2-D)
  Reshape2 : Reshape  OutputDimensionality=Row vector (2-D)
  Selector6 : Selector  InputPortWidth=17  IndexOptions=Index vector (dialog)  Indices=[4]  OutputSizes=1
  Gyroscopic moment [Body axes] : Outport
  wires:
  Body_rates/1 -> Reshape2/1
  Product5/1 -> Reshape1/1
  Cross Product/1(u x v) -> Product5/3
  Propeller moment of inertia/1(Out1) -> Product5/1  "Moment of inertia for each propeller"
  Selector6/1 -> Product5/2  "Direction of propeller rotation (+1 for CW, -1 for CCW)"
  Conversion rpm to rad/s/1 -> Product5/4
  RPM_motor/1 -> Conversion rpm to rad/s/1
  MotorMatrix_real/1 -> Selector6/1, Propeller moment of inertia/1(In1)
  Thrust_direction (Body axes)/1 -> Cross Product/2(v)  "Thrust direction (Body axes)"
  Reshape2/1 -> Cross Product/1(u)
  Reshape1/1 -> Gyroscopic moment [Body axes]/1
